simulink model "DampingAnalysis_Integration_TestModel"  (R2014a)
settings: Solver=ode8  StartTime=0.0  StopTime=10.0  FixedStep=0.01  RelTol=1e-3
undefined symbols (not defined in the file or in its folder): initial_disturbance
libraries: rocket_angular_flight_library x6
settings Model: Creator=scorpii  LastModifiedBy=scorpii

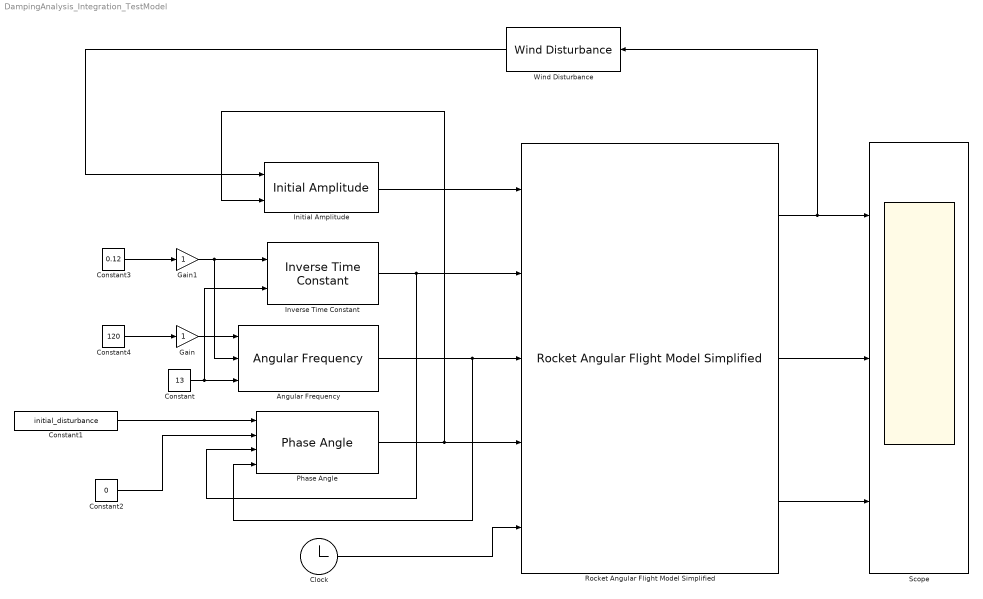
== system DampingAnalysis_Integration_TestModel ==
  Angular Frequency : rocket_angular_flight_library/Angular Frequency
  Clock : Clock
  Constant : Constant  Value=13
  Constant1 : Constant  Value=initial_disturbance
  Constant2 : Constant  Value=0
  Constant3 : Constant  Value=0.12
  Constant4 : Constant  Value=120
  Gain : Gain
  Gain1 : Gain
  Initial Amplitude : rocket_angular_flight_library/Initial Amplitude
  Inverse Time Constant : rocket_angular_flight_library/Inverse Time Constant
  Phase Angle : rocket_angular_flight_library/Phase Angle
  Rocket Angular Flight Model Simplified : rocket_angular_flight_library/Rocket Angular Flight Model Simplified  SystemSampleTime=-1
  Scope : Scope  NumInputPorts=3
      settings: YMin=-5~-5~-5  YMax=5~5~5
  Wind Disturbance : rocket_angular_flight_library/Wind Disturbance
  wires:
  Initial Amplitude/1 -> Rocket Angular Flight Model Simplified/1
  Inverse Time Constant/1 -> Rocket Angular Flight Model Simplified/2, Phase Angle/3
  Angular Frequency/1 -> Rocket Angular Flight Model Simplified/3, Phase Angle/4
  Phase Angle/1 -> Initial Amplitude/2, Rocket Angular Flight Model Simplified/4
  Clock/1 -> Rocket Angular Flight Model Simplified/5
  Rocket Angular Flight Model Simplified/1 -> Wind Disturbance/1, Scope/1
  Constant4/1 -> Gain/1
  Gain/1 -> Angular Frequency/1
  Gain1/1 -> Angular Frequency/2, Inverse Time Constant/1
  Rocket Angular Flight Model Simplified/2 -> Scope/2
  Constant/1 -> Angular Frequency/3, Inverse Time Constant/2
  Rocket Angular Flight Model Simplified/3 -> Scope/3
  Wind Disturbance/1 -> Initial Amplitude/1
  Constant2/1 -> Phase Angle/2
  Constant1/1 -> Phase Angle/1
  Constant3/1 -> Gain1/1
